simulink model "test_lab"  (Simulink 7.7)
settings: Solver=ode45  StartTime=0.0  StopTime=Tt  RelTol=1e-3
undefined symbols (not defined in the file): a, b, c, K, r
settings Model: Creator=pdoren  LastModifiedBy=pdoren  CovModelRefEnable=off
settings SolverCC: ZeroCrossAlgorithm=Adaptive
settings DataIOCC: SaveFormat=StructureWithTime  SignalLoggingSaveFormat=Dataset
settings OptimizationCC: ExpressionDepthLimit=128
settings DebuggingCC: UnderspecifiedInitializationDetection=Simplified  MergeDetectMultiDrivingBlocksExec=error  SolverPrmCheckMsg=none  FcnCallInpInsideContextMsg=Enable All  StateNameClashWarn=none
settings HardwareCC: ProdBitPerPointer=64  ProdLargestAtomicFloat=Float  ProdIntDivRoundTo=Zero  ProdEndianess=LittleEndian  ProdHWDeviceType=Specified
settings CodeAppCC: CustomSymbolStrType=$N$R$M_T
settings GRTTargetCC: TargetFunctionLibrary=C89/C90 (ANSI)  GeneratePreprocessorConditionals=Use local settings

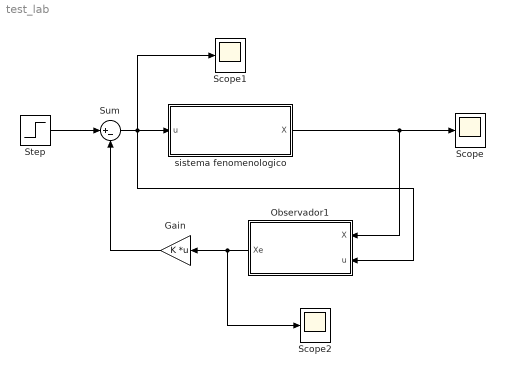
== system test_lab ==
  Gain : Gain  Gain=K  Multiplication=Matrix(K*u)
  Observador1 : Subsystem
  Scope : Scope
      settings: TimeRange=auto  MaxDataPoints=5000  SaveName=estados_observados  YMin=-0.0244  YMax=0.0253  SampleTime=-1  DataFormat=Array
  Scope1 : Scope
      settings: TimeRange=auto  MaxDataPoints=5000  SaveName=entrada  YMin=-4973506511820882200000000000000000000000000000000000000000000000000000000000000000000000000000.00000  YMax=1962907007491516200000000000000000000000000000000000000000000000000000000000000000000000000000.00000  SampleTime=-1  DataFormat=Array
  Scope2 : Scope
      settings: TimeRange=auto  MaxDataPoints=5000  SaveName=estados_estimados  YMin=-4973506511820882200000000000000000000000000000000000000000000000000000000000000000000000000000.00000  YMax=1962907007491516200000000000000000000000000000000000000000000000000000000000000000000000000000.00000  SampleTime=-1  DataFormat=Array
  Step : Step  After=r  SampleTime=0
  Sum : Sum  Inputs=|+-
  sistema fenomenologico : Subsystem
  wires:
  Sum/1 -> Scope1/1, Observador1/2(u), sistema fenomenologico/1(u)
  Step/1 -> Sum/1
  Gain/1 -> Sum/2
  sistema fenomenologico/1(X) -> Observador1/1(X), Scope/1
  Observador1/1(Xe) -> Gain/1, Scope2/1

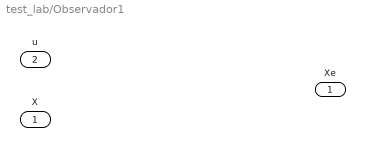
== system test_lab/Observador1 ==
  X : Inport
  u : Inport  Port=2
  Xe : Outport

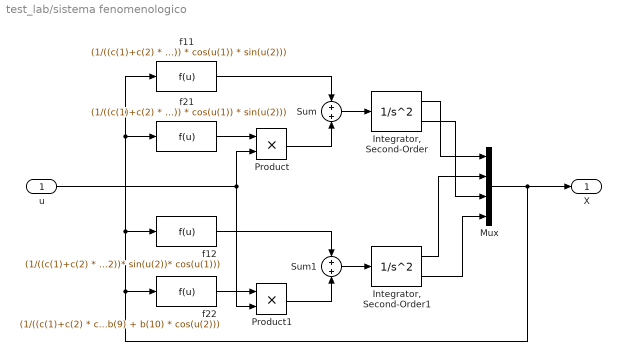
== system test_lab/sistema fenomenologico ==
  u : Inport
  "Integrator, Second-Order" : SecondOrderIntegrator  ICX=x1  ICDXDT=x3
  "Integrator, Second-Order1" : SecondOrderIntegrator  ICX=x2  ICDXDT=x4
  Mux : Mux
  Product : Product
  Product1 : Product
  Sum : Sum  Inputs=+|+
  Sum1 : Sum  Inputs=+|+
  f11 : Fcn  Expr=(1/((c(1)+c(2) * cos(u(2))^2) * c(3))) * ((a(1) + a(2) * cos(u(2))) * sin(u(2)) * u(3)^2 + a(3) * sin(u(2)) * u(4) * u(3) + a(4) * sin(u(2)) * u(4)^2 + (a(5) + a(6) * cos(u(2))) * u(4) + a(9) * sin(u(1)) * cos(u(2))^2 + a(10) * sin(u(1)) + a(11) * cos(u(2)) * cos(u(1)) * sin(u(2)))
  f12 : Fcn  Expr=(1/((c(1)+c(2) * cos(u(2))^2) * c(3))) * ((b(1) + b(2) * cos(u(2))) * sin(u(2)) * u(3)^2 + (b(3) * cos(u(2)) + b(4))* sin(u(2)) * u(4) * u(1) + (b(5) + b(6) * cos(u(2)))* sin(u(2)) * u(4)^2 + (b(7) + b(8)* cos(u(2))) * u(4) + (b(11) + b(12)* cos(u(2)))* sin(u(1)) + b(13) * sin(u(1)) * cos(u(2))^2 + b(14) * cos(u(1)) * sin(u(2)) + b(15) * cos(u(2))* sin(u(2))* cos(u(1)))
  f21 : Fcn  Expr=(1/((c(1)+c(2) * cos(u(2))^2) * c(3))) * ((a(1) + a(2) * cos(u(2))) * sin(u(2)) * u(3)^2 + a(3) * sin(u(2)) * u(4) * u(3) + a(4) * sin(u(2)) * u(4)^2 + (a(5) + a(6) * cos(u(2))) * u(4) + a(9) * sin(u(1)) * cos(u(2))^2 + a(10) * sin(u(1)) + a(11) * cos(u(2)) * cos(u(1)) * sin(u(2)))
  f22 : Fcn  Expr=(1/((c(1)+c(2) * cos(u(2))^2) * c(3))) * (b(9) + b(10) * cos(u(2)))
  X : Outport
  wires:
  Product/1 -> Sum/2
  f11/1 -> Sum/1
  f21/1 -> Product/1
  "Integrator, Second-Order"/1 -> Mux/1
  "Integrator, Second-Order1"/2 -> Mux/4
  Sum1/1 -> "Integrator, Second-Order1"/1
  "Integrator, Second-Order"/2 -> Mux/3
  "Integrator, Second-Order1"/1 -> Mux/2
  u/1 -> Product1/2, Product/2
  Mux/1 -> X/1, f22/1, f12/1, f21/1, f11/1
  Sum/1 -> "Integrator, Second-Order"/1
  f12/1 -> Sum1/1
  f22/1 -> Product1/1
  Product1/1 -> Sum1/2
